simulink model "aubo_robot"  (R2025b)
settings: Solver=ode4  StartTime=0.0  StopTime=10.0  FixedStep=0.005  MaxStep=0.2  RelTol=1e-3
PostLoadFcn:
  | rigid_body = importrobot('urdf\aubo_description\urdf\aubo_i5.urdf');
  | rigid_body.DataFormat = 'column';
  | rigid_body.Gravity = [0 0 -9.81];
  | init_joint_pos = [0,-45,90,45,90, 0] / 180 * pi;
  | robot = get_robot_chain(rigid_body);
  | n = robot.dof;
  | T_init = forward_kin_general(robot, init_joint_pos);
undefined symbols (not defined in the file or in its folder): trvec2tform
libraries: my_library x3, robotcorelib x2
settings Model: Creator=Junch  LastModifiedBy=Junch

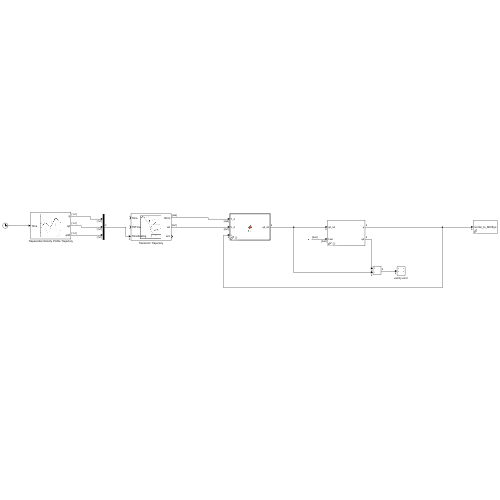
[thumbnail: Simulink's stored preview of the top-level diagram]
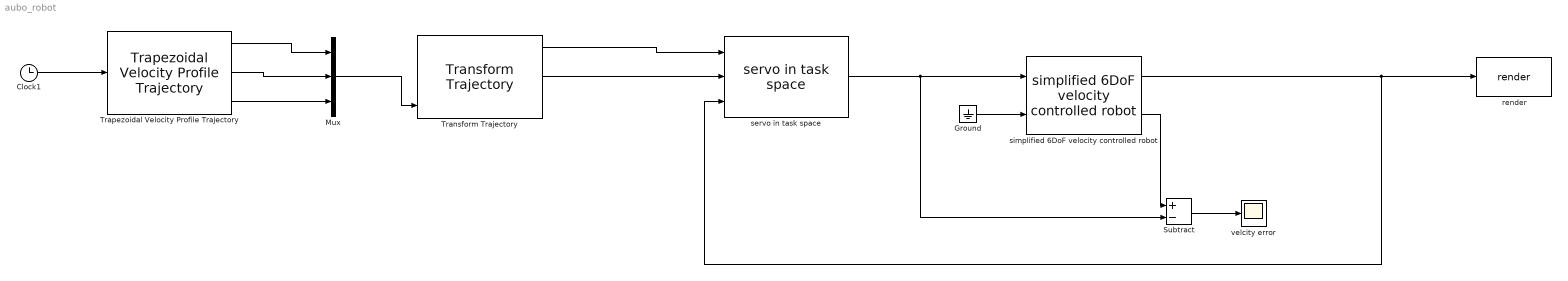
== system aubo_robot ==
  Clock1 : Clock
  Ground : Ground
  Mux : Mux  Inputs=3
  Subtract : Sum  Inputs=+-
  Transform Trajectory : robotcorelib/Transform Trajectory  WaypointSource=Internal  T0=T_init  TF=T_init * trvec2tform( [ 0, 0, -0.25 ] )  TimeInterval=[0, 1]  CustomTimeScaling=on  ParameterSource=External  TSTime=2:0.1:3  TimeScaling=[ 0:0.1:1; ones( 1, 11 ); zeros( 1, 11 ) ]  SimulateUsing=Interpreted execution
      settings: LibrarySourceBlock=robotutilslib/Transform Trajectory
  Trapezoidal Velocity Profile Trajectory : robotcorelib/Trapezoidal Velocity Profile Trajectory  WaypointSource=Internal  Waypoints=[ 0, 1]  NumParams=1  Parameter1=End Time  Parameter2=End Time  ParameterSource=Internal  PeakVelocity=[ 2; 2 ]  Acceleration=[ 1; 2 ]  EndTime=10  AccelTime=[ 1; 2 ]  SimulateUsing=Interpreted execution
  render : my_library/render  Ts=0.05
      settings: SourceProductName=MyLibrary
  servo in task space : my_library/servo in task space  robot=robot  Kp=10 * ones(1, 6)  threshold=5000  lambda=0.1
  simplified 6DoF velocity controlled robot : my_library/simplified 6DoF velocity controlled robot  robot=robot  q0=init_joint_pos
      settings: SourceProductName=MyLibrary
  velcity error : Scope
      settings: ActiveDisplayYMinimum=-0.0035574663624260974  ActiveDisplayYMaximum=0.00406429240754507  DataLoggingVariableName=ScopeData3
  wires:
  simplified 6DoF velocity controlled robot/2 -> Subtract/1
  simplified 6DoF velocity controlled robot/1 -> servo in task space/3, render/1
  Clock1/1 -> Trapezoidal Velocity Profile Trajectory/1
  Transform Trajectory/1 -> servo in task space/1
  Transform Trajectory/2 -> servo in task space/2
  Subtract/1 -> velcity error/1
  Trapezoidal Velocity Profile Trajectory/1 -> Mux/1
  Trapezoidal Velocity Profile Trajectory/2 -> Mux/2
  Mux/1 -> Transform Trajectory/3
  servo in task space/1 -> simplified 6DoF velocity controlled robot/1, Subtract/2
  Trapezoidal Velocity Profile Trajectory/3 -> Mux/3
  Ground/1 -> simplified 6DoF velocity controlled robot/2
